simulink model "model"  (Simulink 8.2)
settings: Solver=FixedStepDiscrete  StartTime=0.0  StopTime=50  RelTol=1e-3
libraries: simulink x2
settings Model: Creator=Toni  LastModifiedBy=Toni
settings DataIOCC: SignalLoggingSaveFormat=Dataset
settings OptimizationCC: ExpressionDepthLimit=128
settings DebuggingCC: FcnCallInpInsideContextMsg=EnableAllAsError  StateNameClashWarn=none
settings GRTTargetCC: CombineOutputUpdateFcns=on  GRTInterface=off

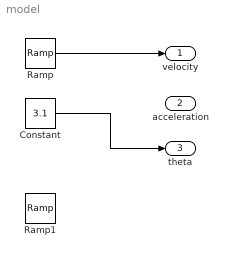
== system model ==
  Constant : Constant  Value=3.1
  Ramp : simulink/Sources/Ramp  slope=1  start=0  X0=0
  Ramp1 : simulink/Sources/Ramp  slope=3.1/100  start=0  X0=0
  velocity : Outport
  acceleration : Outport  Port=2
  theta : Outport  Port=3
  wires:
  Constant/1 -> theta/1
  Ramp/1 -> velocity/1
